simulink model "STGexample"  (R2022a)
settings: Solver=VariableStepAuto  StartTime=0.0  StopTime=10.0  RelTol=1e-3
libraries: neuromorphic_blocks x8
settings Model: Creator=chris  LastModifiedBy=chris

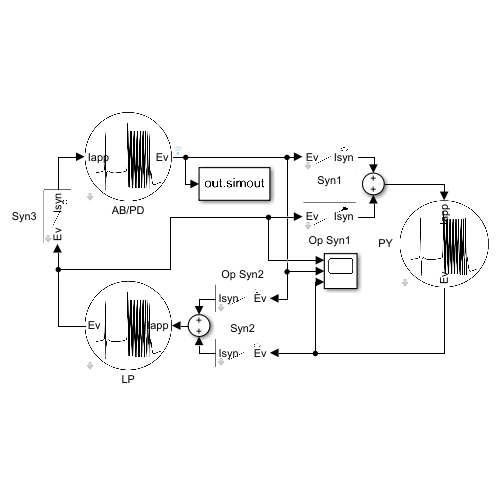
[thumbnail: Simulink's stored preview of the top-level diagram]
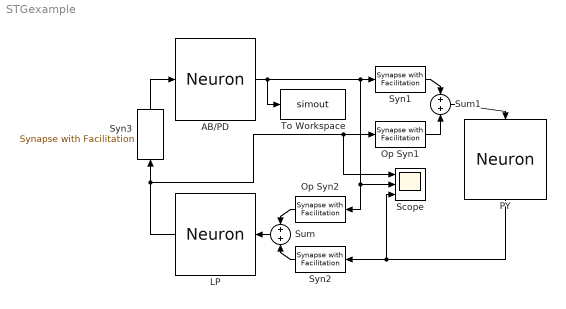
== system STGexample ==
  AB/PD : neuromorphic_blocks/Neural Blocks/Neuron  gfm_source=Internal  gfm=2  gsp_source=Internal  gsp=4  gsm_source=Internal  gsm=2  gup_source=Internal  gup=1.5  gum_source=Internal  gum=0  dfm=0  dsp=0.5  dsm=-0.5  dup=-0.5  dum=-1  mfm=1  msp=1  msm=1  mup=1  mum=1  timescale=0.004  rel_membrane=0.1  rel_fast=0.1  rel_slow=3.1623  rel_ultraslow=100  Iapp_base=0.15  V0=-1.2  tresh=0  output=Events
      settings: SourceProductName=NeurCont Toolbox
  LP : neuromorphic_blocks/Neural Blocks/Neuron  gfm_source=Internal  gfm=2  gsp_source=Internal  gsp=4  gsm_source=Internal  gsm=2  gup_source=Internal  gup=1.5  gum_source=Internal  gum=0  dfm=0  dsp=0.5  dsm=-0.5  dup=-0.5  dum=-1  mfm=1  msp=1  msm=1  mup=1  mum=1  timescale=0.004  rel_membrane=0.1  rel_fast=0.1  rel_slow=3.1623  rel_ultraslow=100  Iapp_base=0.15  V0=-1.2  tresh=0  output=Events
      settings: SourceProductName=NeurCont Toolbox
  Op Syn1 : neuromorphic_blocks/Neural Blocks/Synapse with Facilitation  gsyn_source=Internal  gsyn=1.2  dsyn=4  msyn=10  timescale=0.004  rel_timescale=10  input=Events  gsyn_in=0  dsyn_in=0  msyn_in=1
      settings: SourceProductName=NeurCont Toolbox
  Op Syn2 : neuromorphic_blocks/Neural Blocks/Synapse with Facilitation  gsyn_source=Internal  gsyn=-1  dsyn=4  msyn=10  timescale=0.004  rel_timescale=10  input=Events  gsyn_in=0  dsyn_in=0  msyn_in=1
      settings: SourceProductName=NeurCont Toolbox
  PY : neuromorphic_blocks/Neural Blocks/Neuron  gfm_source=Internal  gfm=2  gsp_source=Internal  gsp=4  gsm_source=Internal  gsm=2  gup_source=Internal  gup=1.5  gum_source=Internal  gum=0  dfm=0  dsp=0.5  dsm=-0.5  dup=-0.5  dum=-1  mfm=1  msp=1  msm=1  mup=1  mum=1  timescale=0.004  rel_membrane=0.1  rel_fast=0.1  rel_slow=3.1623  rel_ultraslow=100  Iapp_base=0.15  V0=-1.2  tresh=0  output=Events
      settings: SourceProductName=NeurCont Toolbox
  Scope : Scope  NumInputPorts=3
  Sum : Sum  Inputs=+|+
  Sum1 : Sum  Inputs=+|+
  Syn1 : neuromorphic_blocks/Neural Blocks/Synapse with Facilitation  gsyn_source=Internal  gsyn=-0.9  dsyn=4  msyn=10  timescale=0.004  rel_timescale=10  input=Events  gsyn_in=0  dsyn_in=0  msyn_in=1
      settings: SourceProductName=NeurCont Toolbox
  Syn2 : neuromorphic_blocks/Neural Blocks/Synapse with Facilitation  gsyn_source=Internal  gsyn=-0.5  dsyn=4  msyn=10  timescale=0.004  rel_timescale=10  input=Events  gsyn_in=0  dsyn_in=0  msyn_in=1
      settings: SourceProductName=NeurCont Toolbox
  Syn3 : neuromorphic_blocks/Neural Blocks/Synapse with Facilitation  gsyn_source=Internal  gsyn=-0.2  dsyn=4  msyn=10  timescale=0.004  rel_timescale=10  input=Events  gsyn_in=0  dsyn_in=0  msyn_in=1
      settings: SourceProductName=NeurCont Toolbox
  To Workspace : ToWorkspace  VariableName=simout  SaveFormat=Timeseries  SampleTime=-1
  wires:
  Sum/1 -> LP/1
  Syn2/1 -> Sum/2
  Op Syn2/1 -> Sum/1
  Op Syn1/1 -> Sum1/2
  Syn1/1 -> Sum1/1
  Sum1/1 -> PY/1
  LP/1 -> Syn3/1, Scope/1, Op Syn1/1
  Syn3/1 -> AB/PD/1
  AB/PD/1 -> Scope/2, Op Syn2/1, Syn1/1, To Workspace/1
  PY/1 -> Scope/3, Syn2/1
